simulink model "Project7"  (R2018b)
settings: Solver=ode4  StartTime=0.0  StopTime=1e-4  FixedStep=10e-12  RelTol=1e-3
libraries: simulink x2
settings Model: Creator=Samjat Chan  LastModifiedBy=Samjat Chan

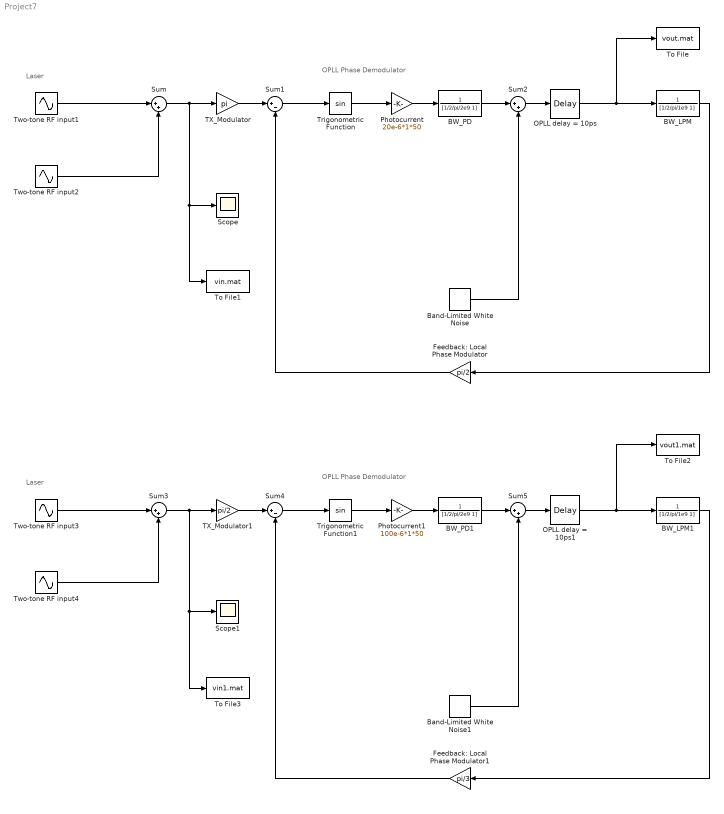
== system Project7 ==
  note: OPLL Phase Demodulator
  note: Laser
  note: OPLL Phase Demodulator
  note: Laser
  BW_LPM : TransferFcn  Denominator=[1/2/pi/1e9 1]
  BW_LPM1 : TransferFcn  Denominator=[1/2/pi/1e9 1]
  BW_PD : TransferFcn  Denominator=[1/2/pi/2e9 1]
  BW_PD1 : TransferFcn  Denominator=[1/2/pi/2e9 1]
  Band-Limited White Noise : simulink/Sources/Band-Limited White Noise  Cov=[(6e-16)/2]  Ts=10e-12  seed=[23341]
  Band-Limited White Noise1 : simulink/Sources/Band-Limited White Noise  Cov=[(6e-16)/2]  Ts=10e-12  seed=[23341]
  Feedback: Local Phase Modulator : Gain  Gain=pi/2
  Feedback: Local Phase Modulator1 : Gain  Gain=pi/3
  OPLL delay = 10ps : TransportDelay  DelayTime=10e-12  BufferSize=1024*16
  OPLL delay = 10ps1 : TransportDelay  DelayTime=10e-12  BufferSize=1024*16
  Photocurrent : Gain  Gain=20e-6*1*50
  Photocurrent1 : Gain  Gain=100e-6*1*50
  Scope : Scope
  Scope1 : Scope
  Sum{,2..3,5} (4 alike) : Sum  Inputs=|++
  Sum1 : Sum  Inputs=|+-
  Sum4 : Sum  Inputs=|+-
  TX_Modulator : Gain  Gain=pi
  TX_Modulator1 : Gain  Gain=pi/2
  To File : ToFile  Filename=vout.mat  MatrixName=vout
  To File1 : ToFile  Filename=vin.mat  MatrixName=vin
  To File2 : ToFile  Filename=vout1.mat  MatrixName=vout1
  To File3 : ToFile  Filename=vin1.mat  MatrixName=vin1
  Trigonometric Function : Trigonometry
  Trigonometric Function1 : Trigonometry
  Two-tone RF input1 : Sin  Amplitude=0.1  Frequency=(2*pi)*(500e6+10e6)  SampleTime=10e-12
  Two-tone RF input2 : Sin  Amplitude=0.1  Frequency=(2*pi)*(500e6-10e6)  SampleTime=10e-12
  Two-tone RF input3 : Sin  Amplitude=0.3  Frequency=(2*pi)*(500e6+10e6)  SampleTime=10e-12
  Two-tone RF input4 : Sin  Amplitude=0.3  Frequency=(2*pi)*(500e6-10e6)  SampleTime=10e-12
  wires:
  Sum/1 -> To File1/1, Scope/1, TX_Modulator/1
  TX_Modulator/1 -> Sum1/1
  Two-tone RF input1/1 -> Sum/1
  Two-tone RF input2/1 -> Sum/2
  OPLL delay = 10ps/1 -> To File/1, BW_LPM/1
  Feedback: Local Phase Modulator/1 -> Sum1/2
  Photocurrent/1 -> BW_PD/1
  BW_LPM/1 -> Feedback: Local Phase Modulator/1
  Sum1/1 -> Trigonometric Function/1
  Sum2/1 -> OPLL delay = 10ps/1
  Band-Limited White Noise/1 -> Sum2/2
  BW_PD/1 -> Sum2/1
  Trigonometric Function/1 -> Photocurrent/1
  Feedback: Local Phase Modulator1/1 -> Sum4/2
  BW_PD1/1 -> Sum5/1
  BW_LPM1/1 -> Feedback: Local Phase Modulator1/1
  Sum5/1 -> OPLL delay = 10ps1/1
  OPLL delay = 10ps1/1 -> To File2/1, BW_LPM1/1
  Sum3/1 -> To File3/1, Scope1/1, TX_Modulator1/1
  Two-tone RF input3/1 -> Sum3/1
  Sum4/1 -> Trigonometric Function1/1
  Photocurrent1/1 -> BW_PD1/1
  Two-tone RF input4/1 -> Sum3/2
  Band-Limited White Noise1/1 -> Sum5/2
  TX_Modulator1/1 -> Sum4/1
  Trigonometric Function1/1 -> Photocurrent1/1
